simulink subsystem "edge2x1_toggleable_asSubsystem"  (R2021a)
settings: Solver=VariableStepAuto  StartTime=0.0  StopTime=10.0  RelTol=1e-3
libraries: EdgesLibrary x2
settings Model: Creator=phill  LastModifiedBy=phill

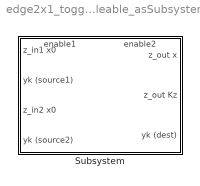
== system edge2x1_toggleable_asSubsystem ==
  Subsystem : Subsystem  mask{Rk1=0, Rk2=0.5}
      mask prompts: Rk1 "Rk (input 1)"; Rk2 "Rk (input 2)"
      settings: PortSchema="{\"entries\":[{\"content\":{\"sides\":[{\"content\":{\"connectorIds\":[\"In1\",\"Out2\",\"In2\",\"Out3\"]},\"type\":\"ConnectorPlacement.EquallySpacedRectSide\",\"uuid\":\"2e9f11d3-65d9-473f-b826-57e0db4d0b8d\"},{\"content\":{\"connectorIds\":[\"In5\",\"In6\",\"Out1\"],\"side\":\"RIGHT\"},\"type\":\"ConnectorPlacement.EquallySpacedRectSide\",\"uuid\":\"d8eabf6d-fb3a-4c3e-97ce-4f99fedc7242\"},{\"content\":{\"connectorIds\":[\"In3\",\"In4\"],\"side\":\"TOP\"},\"type\":\"ConnectorPlacement.EquallySpacedRectSide\",\"uuid\":\"c1317a9d-7aa4-490c-a27e-f3fa93a0d151\"}]},\"type\":\"ConnectorPlacement.EquallySpacedConnector\",\"uuid\":\"3cd892e4-da09-4624-b831-53c46896b420\"}],\"packageUris\":[\"http://schema.mathworks.com/mf0/Connector/R2020b\"],\"version\":\"1.0\"}"
      mask Display:
      | image('$imagefile'); % Use "Edit Image" on toolstrip to change.
      | disp('Toggleable Edge 2x1 \n\n');
      | Rk1 = get_param(gcb,'Rk1');
      | Rk2 = get_param(gcb, 'Rk2');
      | disp(['Rk1 = ', Rk1, ' | Rk2 =  ', Rk2])

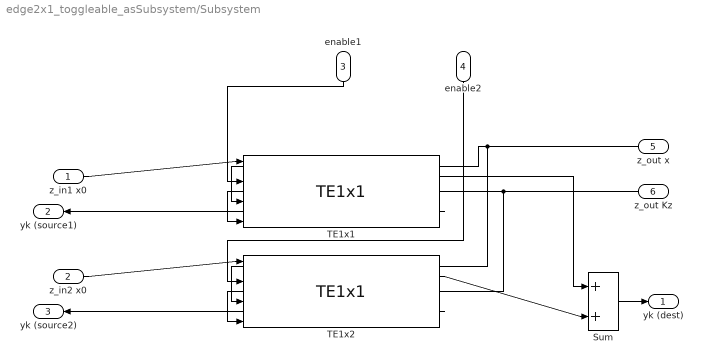
== system edge2x1_toggleable_asSubsystem/Subsystem ==
  z_in1 x0 : Inport
  z_in2 x0 : Inport  Port=2
  enable1 : Inport  Port=3
  enable2 : Inport  Port=4
  z_out x : Inport  Port=5
  z_out Kz : Inport  Port=6
  Sum : Sum
  TE1x1 : EdgesLibrary/TE1x1  Rk=Rk1
  TE1x2 : EdgesLibrary/TE1x1  Rk=Rk2
  yk (dest) : Outport
  yk (source1) : Outport  Port=2
  yk (source2) : Outport  Port=3
  wires:
  Sum/1 -> yk (dest)/1
  z_out x/1 -> TE1x1/3, TE1x2/3
  TE1x2/1 -> Sum/2
  z_in2 x0/1 -> TE1x2/1
  z_out Kz/1 -> TE1x1/4, TE1x2/4
  TE1x1/1 -> Sum/1
  enable2/1 -> TE1x2/2
  enable1/1 -> TE1x1/2
  TE1x2/2 -> yk (source2)/1
  z_in1 x0/1 -> TE1x1/1
  TE1x1/2 -> yk (source1)/1
